simulink model "ar07_mot_03_sim1"  (R2022b)
settings: Solver=ode45  StartTime=0.0  StopTime=100  FixedStep=SIMstepSize  MaxStep=0.02  RelTol=1e-3  EnableMultiTasking=on
values from neighbouring files (symbols this model uses):
  data_Ts = 0.02    [ar07_mot_03_ident.m]
  ok_u_PB = 10    [ar07_mot_03_ident.m]
  u_PB1 = 210    [ar07_mot_03_ident.m]
  u_PB2 = 130    [ar07_mot_03_ident.m]
undefined symbols (not defined in the file or in its folder): pModelKoef, T1pModelKoef, T2pModelKoef
settings Model: Creator=MT  LastModifiedBy=MT
settings SolverCC: AlgebraicLoopSolver=TrustRegion
settings DataIOCC: LimitDataPoints=on  SaveFormat=Array  SignalLoggingSaveFormat=ModelDataLogs  SaveOutput=off  SignalLogging=off  DSMLogging=off  SaveTime=off  ReturnWorkspaceOutputs=off
settings OptimizationCC: ExpressionDepthLimit=2147483647  LifeSpan=inf
settings DebuggingCC: UnderspecifiedInitializationDetection=Classic  MergeDetectMultiDrivingBlocksExec=none  SolverPrmCheckMsg=warning  FcnCallInpInsideContextMsg=warning  UnconnectedInputMsg=warning  UnconnectedOutputMsg=warning  UnconnectedLineMsg=warning  StateNameClashWarn=warning  SFUnexpectedBacktrackingDiag=warning  SFNoUnconditionalDefaultTransitionDiag=warning  SFExecutionAtInitializationDiag=none  SFMachineParentedDataDiag=warning  ArithmeticOperatorsInVariantConditions=warning
settings HardwareCC: ProdBitPerPointer=32  ProdBitPerSizeT=32  ProdBitPerPtrDiffT=32  ProdLargestAtomicFloat=None  ProdIntDivRoundTo=Undefined  ProdEndianess=Unspecified  ProdWordSize=32  ProdHWDeviceType=32-bit Generic
settings ModelReferenceCC: EnableRefExpFcnMdlSchedulingChecks=on  PropagateSignalLabelsOutOfModel=off
settings SFSimCC: SimUseLocalCustomCode=off  CustomCodeUndefinedFunction=UseInterfaceOnly
settings RTWCC: RTWUseLocalCustomCode=off  DLArmComputeVersion=19.05
settings CodeAppCC: StateflowObjectComments=on
settings GRTTargetCC: TargetLangStandard=C89/C90 (ANSI)  CombineOutputUpdateFcns=off  GRTInterface=on
settings ConfigComp: CovMetricSettings=dw  CovSaveCumulativeToWorkspaceVar=on  CovSaveSingleToWorkspaceVar=on  CovExternalEMLEnable=off

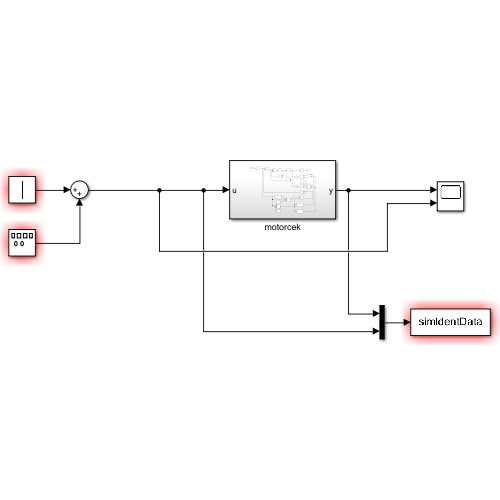
[thumbnail: Simulink's stored preview of the top-level diagram]
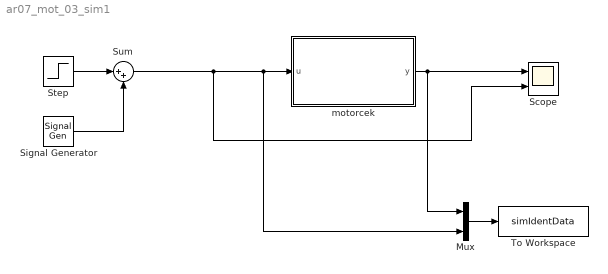
== system ar07_mot_03_sim1 ==
  Mux : Mux  Inputs=2
  Scope : Scope  NumInputPorts=2
  Signal Generator : SignalGenerator  WaveForm=square  Amplitude=-ok_u_PB  Frequency=1/10
  Step : Step  Time=50  Before=u_PB1  After=u_PB2  SampleTime=0
  Sum : Sum  Inputs=|++
  To Workspace : ToWorkspace  VariableName=simIdentData  SaveFormat=Timeseries  SampleTime=data_Ts
  motorcek : Subsystem
  wires:
  Step/1 -> Sum/1
  Sum/1 -> Scope/2, motorcek/1(u), Mux/2
  Signal Generator/1 -> Sum/2
  motorcek/1(y) -> Mux/1, Scope/1
  Mux/1 -> To Workspace/1

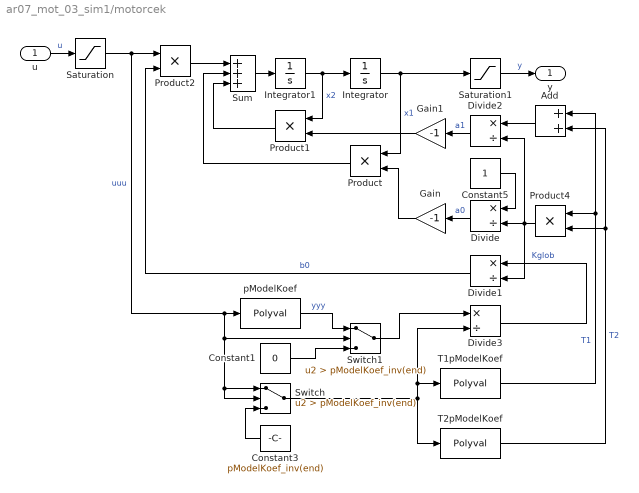
== system ar07_mot_03_sim1/motorcek ==
  u : Inport
  Add : Sum
  Constant1 : Constant  Value=0
  Constant3 : Constant  Value=pModelKoef_inv(end)
  Constant5 : Constant
  Divide{,1..3} (4 alike) : Product  Inputs=*/
  Gain : Gain  Gain=-1
  Gain1 : Gain  Gain=-1
  Integrator : Integrator
  Integrator1 : Integrator
  Product{,1..2,4} (4 alike) : Product
  Saturation : Saturate  UpperLimit=255  LowerLimit=0
  Saturation1 : Saturate  UpperLimit=1023  LowerLimit=0
  Sum : Sum  Inputs=+++
  Switch : Switch  Criteria=u2 > Threshold  Threshold=pModelKoef_inv(end)  SaturateOnIntegerOverflow=off  InputSameDT=off
  Switch1 : Switch  Criteria=u2 > Threshold  Threshold=pModelKoef_inv(end)  SaturateOnIntegerOverflow=off  InputSameDT=off
  T1pModelKoef : Polyval  Coefs=T1pModelKoef
  T2pModelKoef : Polyval  Coefs=T2pModelKoef
  pModelKoef : Polyval  Coefs=pModelKoef
  y : Outport
  wires:
  Gain/1 -> Product/2
  Saturation/1 -> Product2/1, pModelKoef/1, Switch/2, Switch/1, Switch1/2  "uuu"
  Product1/1 -> Sum/3
  Sum/1 -> Integrator1/1
  Product4/1 -> Divide1/2, Divide2/2, Divide/2
  Constant5/1 -> Divide/1
  T1pModelKoef/1 -> Add/1, Product4/1  "T1"
  Integrator/1 -> Saturation1/1, Product/1  "x1"
  Divide1/1 -> Product2/2  "b0"
  T2pModelKoef/1 -> Add/2, Product4/2  "T2"
  Integrator1/1 -> Integrator/1, Product1/1  "x2"
  Product/1 -> Sum/2
  Gain1/1 -> Product1/2
  Divide/1 -> Gain/1  "a0"
  Product2/1 -> Sum/1
  Switch/1 -> T2pModelKoef/1, T1pModelKoef/1, Divide3/2
  Constant3/1 -> Switch/3
  Divide2/1 -> Gain1/1  "a1"
  Add/1 -> Divide2/1
  Saturation1/1 -> y/1  "y"
  u/1 -> Saturation/1  "u"
  Constant1/1 -> Switch1/3
  pModelKoef/1 -> Switch1/1  "yyy"
  Switch1/1 -> Divide3/1
  Divide3/1 -> Divide1/1  "Kglob"
